simulink model "PMSM_SimModel"  (R2018b)
settings: Solver=VariableStepAuto  StartTime=0.0  StopTime=10.0  RelTol=1e-3
libraries: simulink x8, powerlib x5
settings Model: Creator=fei  LastModifiedBy=fei
settings SolverCC: ZeroCrossAlgorithm=Adaptive
settings DebuggingCC: IgnoredZcDiagnostic=none

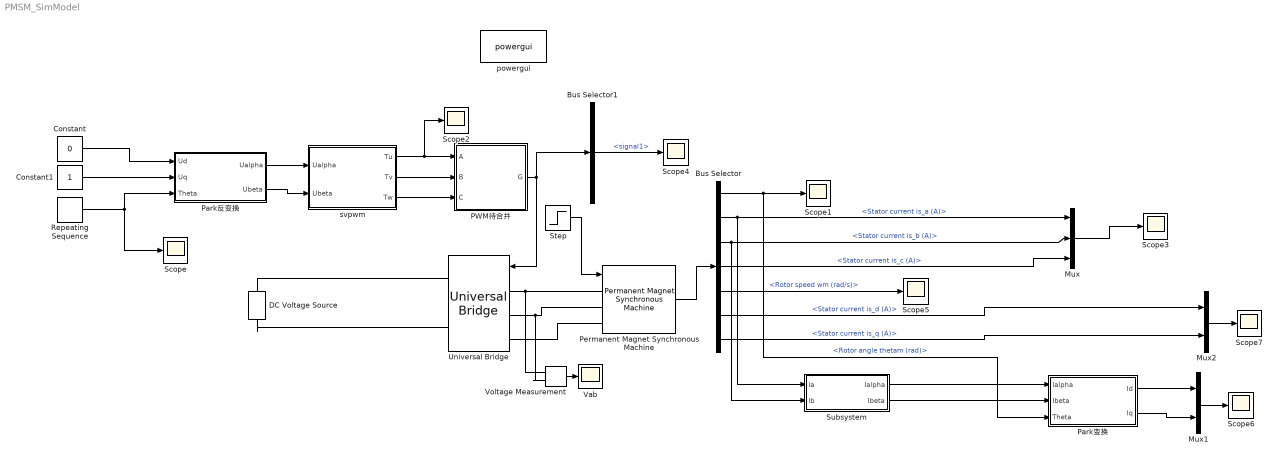
== system PMSM_SimModel ==
  Bus Selector : BusSelector  OutputSignals=Rotor angle thetam (rad),Stator current is_a (A),Stator current is_b (A),Stator current is_c (A),Rotor speed wm (rad/s),Stator current is_d (A),Stator current is_q (A)
  Bus Selector1 : BusSelector  OutputSignals=signal1
  Constant : Constant  Value=0
  Constant1 : Constant
  DC Voltage Source : powerlib/Electrical Sources/DC Voltage Source  Amplitude=48  Measurements=None
  Mux : Mux  Inputs=3
  Mux1 : Mux  Inputs=2
  Mux2 : Mux  Inputs=2
  "PWM待合并 " : Subsystem
  Park反变换 : Subsystem
  Park变换 : Subsystem
  Permanent Magnet Synchronous Machine : powerlib/Machines/Permanent Magnet Synchronous Machine  NbPhases=3  FluxDistribution=Sinusoidal  RotorType=Round  MechanicalLoad=Torque Tm  PresetModel=No  ShowDetailedParameters=on  MeasurementBus=off  Resistance=0.0485  Inductance=8.5e-3  dqInductances=[8.5e-3,8.5e-3]  La=0.000395  MachineConstant=Flux linkage established by magnets (V.s)  Flux=0.1194  VoltageCst=86.6271  TorqueCst=0.7164  Flat=120  Mechanical=[0.0027 0.0004924 4 0]  PolePairs=4  InitialConditions=[0,0, 0,0]  InitialConditions5ph=[0 0 0 0 0 0]  TsPowergui=0  TsBlock=-1  RefAngle=90 degrees behind phase A axis (modified Park)
      settings: SourceProductName=Simscape Power Systems
  Repeating Sequence : simulink/Sources/Repeating Sequence  rep_seq_t=[0 0.5]  rep_seq_y=[0 2*pi]
  Scope{,1..7} (8 alike) : Scope
  Step : Step  SampleTime=0
  Subsystem : Subsystem
  Universal Bridge : powerlib/Power Electronics/Universal Bridge  Arms=3  SnubberResistance=1e5  SnubberCapacitance=inf  Device=MOSFET / Diodes  Ron=1e-3  Lon=0  ForwardVoltages="[  0  0  ]"  ForwardVoltage=0  GTOparameters=[ 10e-6 , 20e-6 ]  IGBTparameters=[ 1e-6 , 2e-6 ]  Measurements=None  Measurements_2=None  converterType=Rectifier
  Vab : Scope
  Voltage Measurement : powerlib/Measurements/Voltage Measurement  PhasorSimulation=off  OutputType=Complex  PSBequivalent=0
      settings: SourceProductName=Simscape Electrical
  powergui : powerlib/powergui  Priority=1  SimulationMode=Continuous  SampleTime=50e-6  frequency=60  Iterations=50  frequencyindice=0  Pbase=100e6  ErrMax=1e-4  UnitsV=kV  UnitsW=MW  buscounter=0  FunctionMessages=off  echomessages=off  EnableUseOfTLC=off  CurrentSourceSwitches=off  DisableSnubberDevices=off  DisableRonSwitches=off  DisableVfSwitches=off  DisplayEquations=off  SolverType=Tustin/Backward Euler (TBE)  Interpol=off  ExternalGateDelay=off  methode=off  Ts=100  x0status=blocks  SPID=on  SwTol=0  HookPort=off  RestoreLinks=warning  ResistiveCurrentMeasurement=off  Frange=[0:2:500]  Ylog=off  Xlog=on  ShowGrid=off  save=off  variable=ZData  structure=0  ZoomFFT=off  StartTime=0.0  cycles=1  DisplayStyle=1  fundamental=60  FreqAxis=off  MaxFrequency=1000  frequencyindicesteady=1  RmsSteady=1  display=off
  svpwm : Subsystem
  wires:
  Constant/1 -> Park反变换/1(Ud)
  Constant1/1 -> Park反变换/2(Uq)
  Repeating Sequence/1 -> Scope/1, Park反变换/3(Theta)
  Park反变换/1(Ualpha) -> svpwm/1(Ualpha)
  Park反变换/2(Ubeta) -> svpwm/2(Ubeta)
  svpwm/1(Tu) -> Scope2/1, "PWM待合并 "/1(A)
  svpwm/2(Tv) -> "PWM待合并 "/2(B)
  svpwm/3(Tw) -> "PWM待合并 "/3(C)
  Step/1 -> Permanent Magnet Synchronous Machine/1
  Voltage Measurement/1 -> Vab/1
  Permanent Magnet Synchronous Machine/1 -> Bus Selector/1
  Bus Selector/1 -> Park变换/3(Theta), Scope1/1  "<Rotor angle thetam (rad)>"
  Bus Selector/2 -> Subsystem/1(Ia), Mux/1  "<Stator current is_a (A)>"
  Bus Selector/3 -> Subsystem/2(Ib), Mux/2  "<Stator current is_b (A)>"
  Bus Selector/4 -> Mux/3  "<Stator current is_c (A)>"
  Mux/1 -> Scope3/1
  "PWM待合并 "/1(G) -> Bus Selector1/1, Universal Bridge/1
  Bus Selector1/1 -> Scope4/1  "<signal1>"
  Bus Selector/5 -> Scope5/1  "<Rotor speed wm (rad/s)>"
  Subsystem/1(Ialpha) -> Park变换/1(Ialpha)
  Subsystem/2("Ibeta ") -> Park变换/2(Ibeta)
  Mux1/1 -> Scope6/1
  Park变换/1(Id) -> Mux1/1
  Park变换/2(Iq) -> Mux1/2
  Bus Selector/7 -> Mux2/2  "<Stator current is_q (A)>"
  Bus Selector/6 -> Mux2/1  "<Stator current is_d (A)>"
  Mux2/1 -> Scope7/1
  connections:
  Universal Bridge/LConn1 -- Voltage Measurement/LConn1 -- Permanent Magnet Synchronous Machine/LConn1
  Universal Bridge/LConn2 -- Voltage Measurement/LConn2 -- Permanent Magnet Synchronous Machine/LConn2
  Universal Bridge/LConn3 -- Permanent Magnet Synchronous Machine/LConn3
  DC Voltage Source/RConn1 -- Universal Bridge/RConn1
  DC Voltage Source/LConn1 -- Universal Bridge/RConn2

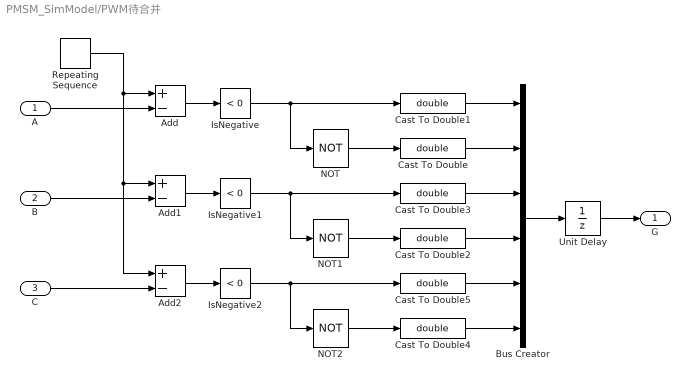
== system PMSM_SimModel/PWM待合并  ==
  A : Inport
  B : Inport  Port=2
  C : Inport  Port=3
  Add : Sum  Inputs=+-
  Add1 : Sum  Inputs=+-
  Add2 : Sum  Inputs=+-
  Bus Creator : BusCreator  Inputs=6
  Cast To Double{,1..5} (6 alike) : DataTypeConversion  OutDataTypeStr=double
  IsNegative : simulink/Logic and Bit Operations/Compare To Zero  relop=<  OutDataTypeStr=boolean
  IsNegative1 : simulink/Logic and Bit Operations/Compare To Zero  relop=<  OutDataTypeStr=boolean
  IsNegative2 : simulink/Logic and Bit Operations/Compare To Zero  relop=<  OutDataTypeStr=boolean
  NOT : Logic  Operator=NOT  IconShape=distinctive  AllPortsSameDT=off  OutDataTypeStr=boolean
  NOT1 : Logic  Operator=NOT  IconShape=distinctive  AllPortsSameDT=off  OutDataTypeStr=boolean
  NOT2 : Logic  Operator=NOT  IconShape=distinctive  AllPortsSameDT=off  OutDataTypeStr=boolean
  Repeating Sequence : simulink/Sources/Repeating Sequence  rep_seq_t=[0 0.0005 0.001]  rep_seq_y=[0 1 0]
  Unit Delay : UnitDelay  SampleTime=-1
  G : Outport
  wires:
  A/1 -> Add/2
  Repeating Sequence/1 -> Add2/1, Add1/1, Add/1
  Add/1 -> IsNegative/1
  IsNegative/1 -> NOT/1, Cast To Double1/1
  NOT/1 -> Cast To Double/1
  NOT1/1 -> Cast To Double2/1
  Add1/1 -> IsNegative1/1
  IsNegative1/1 -> NOT1/1, Cast To Double3/1
  NOT2/1 -> Cast To Double4/1
  Add2/1 -> IsNegative2/1
  IsNegative2/1 -> NOT2/1, Cast To Double5/1
  B/1 -> Add1/2
  C/1 -> Add2/2
  Cast To Double1/1 -> Bus Creator/1
  Cast To Double/1 -> Bus Creator/2
  Cast To Double3/1 -> Bus Creator/3
  Cast To Double2/1 -> Bus Creator/4
  Cast To Double5/1 -> Bus Creator/5
  Cast To Double4/1 -> Bus Creator/6
  Bus Creator/1 -> Unit Delay/1
  Unit Delay/1 -> G/1

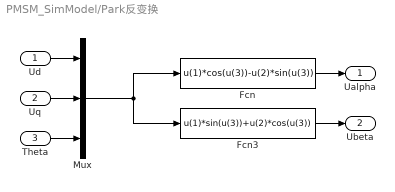
== system PMSM_SimModel/Park反变换 ==
  Ud : Inport
  Uq : Inport  Port=2
  Theta : Inport  Port=3
  Fcn : Fcn  Expr=u(1)*cos(u(3))-u(2)*sin(u(3))
  Fcn3 : Fcn  Expr=u(1)*sin(u(3))+u(2)*cos(u(3))
  Mux : Mux  Inputs=3
  Ualpha : Outport
  Ubeta : Outport  Port=2
  wires:
  Ud/1 -> Mux/1
  Uq/1 -> Mux/2
  Theta/1 -> Mux/3
  Mux/1 -> Fcn3/1, Fcn/1
  Fcn3/1 -> Ubeta/1
  Fcn/1 -> Ualpha/1

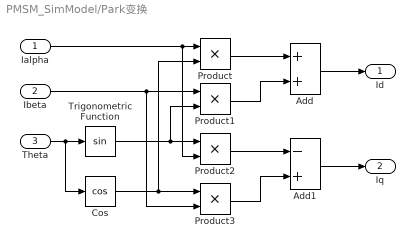
== system PMSM_SimModel/Park变换 ==
  Ialpha : Inport
  Ibeta : Inport  Port=2
  Theta : Inport  Port=3
  Add : Sum
  Add1 : Sum  Inputs=-+
  Cos : Trigonometry  Operator=cos
  Product{,1..3} (4 alike) : Product
  Trigonometric Function : Trigonometry
  Id : Outport
  Iq : Outport  Port=2
  wires:
  Ialpha/1 -> Product2/2, Product/1
  Ibeta/1 -> Product3/2, Product1/1
  Theta/1 -> Cos/1, Trigonometric Function/1
  Trigonometric Function/1 -> Product1/2, Product2/1
  Cos/1 -> Product/2, Product3/1
  Add1/1 -> Iq/1
  Add/1 -> Id/1
  Product/1 -> Add/1
  Product1/1 -> Add/2
  Product2/1 -> Add1/1
  Product3/1 -> Add1/2

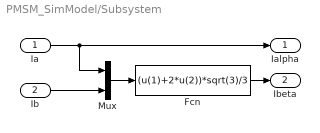
== system PMSM_SimModel/Subsystem ==
  Ia : Inport
  Ib : Inport  Port=2
  Fcn : Fcn  Expr=(u(1)+2*u(2))*sqrt(3)/3
  Mux : Mux  Inputs=2
  Ialpha : Outport
  "Ibeta " : Outport  Port=2
  wires:
  Ia/1 -> Mux/1, Ialpha/1
  Ib/1 -> Mux/2
  Mux/1 -> Fcn/1
  Fcn/1 -> "Ibeta "/1

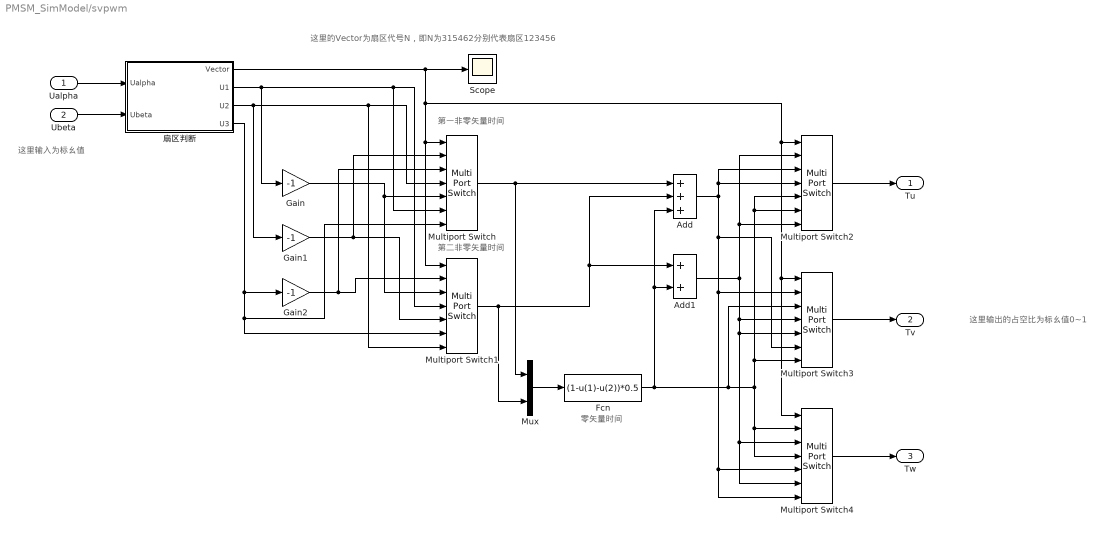
== system PMSM_SimModel/svpwm ==
  note: 这里输出的占空比为标幺值0~1
  note: 这里输入为标幺值
  note: 零矢量时间
  note: 第二非零矢量时间
  note: 第一非零矢量时间
  note: 这里的Vector为扇区代号N，即N为315462分别代表扇区123456
  Ualpha : Inport
  Ubeta : Inport  Port=2
  Add : Sum  Inputs=+++
  Add1 : Sum
  Fcn : Fcn  Expr=(1-u(1)-u(2))*0.5
  Gain : Gain  Gain=-1
  Gain1 : Gain  Gain=-1
  Gain2 : Gain  Gain=-1
  Multiport Switch{,1..4} (5 alike) : MultiPortSwitch  Inputs=6
  Mux : Mux  Inputs=2
  Scope : Scope
  扇区判断 : Subsystem
  Tu : Outport
  Tv : Outport  Port=2
  Tw : Outport  Port=3
  wires:
  Ubeta/1 -> 扇区判断/2(Ubeta)
  Ualpha/1 -> 扇区判断/1(Ualpha)
  扇区判断/1(Vector) -> Multiport Switch3/1, Multiport Switch4/1, Multiport Switch2/1, Multiport Switch1/1, Multiport Switch/1, Scope/1
  扇区判断/2(U1) -> Multiport Switch1/4, Multiport Switch/6, Gain/1
  扇区判断/3(U2) -> Multiport Switch/4, Multiport Switch1/7, Gain1/1
  扇区判断/4(U3) -> Multiport Switch/7, Multiport Switch1/6, Gain2/1
  Gain1/1 -> Multiport Switch1/5, Multiport Switch/2
  Gain2/1 -> Multiport Switch/3, Multiport Switch1/2
  Gain/1 -> Multiport Switch/5, Multiport Switch1/3
  Multiport Switch/1 -> Add/1, Mux/1
  Multiport Switch1/1 -> Add1/1, Add/2, Mux/2
  Mux/1 -> Fcn/1
  Fcn/1 -> Add1/2, Add/3, Multiport Switch4/4, Multiport Switch4/2, Multiport Switch3/7, Multiport Switch2/6, Multiport Switch2/5, Multiport Switch3/3
  Multiport Switch2/1 -> Tu/1
  Multiport Switch3/1 -> Tv/1
  Add1/1 -> Multiport Switch4/6, Multiport Switch4/3, Multiport Switch3/5, Multiport Switch3/4, Multiport Switch2/7, Multiport Switch2/2
  Add/1 -> Multiport Switch2/4, Multiport Switch2/3, Multiport Switch3/6, Multiport Switch4/7, Multiport Switch4/5, Multiport Switch3/2
  Multiport Switch4/1 -> Tw/1

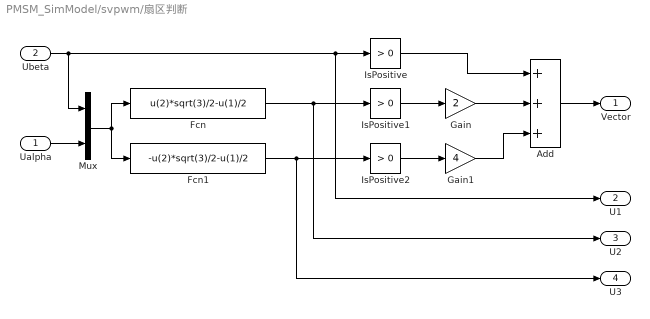
== system PMSM_SimModel/svpwm/扇区判断 ==
  Ualpha : Inport
  Ubeta : Inport  Port=2
  Add : Sum  Inputs=+++
  Fcn : Fcn  Expr=u(2)*sqrt(3)/2-u(1)/2
  Fcn1 : Fcn  Expr=-u(2)*sqrt(3)/2-u(1)/2
  Gain : Gain  Gain=2
  Gain1 : Gain  Gain=4
  IsPositive : simulink/Logic and Bit Operations/Compare To Zero  relop=>  OutDataTypeStr=boolean
  IsPositive1 : simulink/Logic and Bit Operations/Compare To Zero  relop=>  OutDataTypeStr=boolean
  IsPositive2 : simulink/Logic and Bit Operations/Compare To Zero  relop=>  OutDataTypeStr=boolean
  Mux : Mux  Inputs=2
  Vector : Outport
  U1 : Outport  Port=2
  U2 : Outport  Port=3
  U3 : Outport  Port=4
  wires:
  Mux/1 -> Fcn1/1, Fcn/1
  Ualpha/1 -> Mux/2
  IsPositive2/1 -> Gain1/1
  Fcn/1 -> U2/1, IsPositive1/1
  Fcn1/1 -> U3/1, IsPositive2/1
  Gain1/1 -> Add/3
  IsPositive1/1 -> Gain/1
  Gain/1 -> Add/2
  IsPositive/1 -> Add/1
  Add/1 -> Vector/1
  Ubeta/1 -> U1/1, IsPositive/1, Mux/1
